simulink model "LoadLevel3_VF"  (R2023a)
settings: Solver=VariableStepAuto  StartTime=0.0  StopTime=250  RelTol=1e-3
undefined symbols (not defined in the file): a, Ac, Bc, Cc, D1, Dc, Delta, find_system, Fnom, gcbh, I21_init_imag, I21_init_real, Ibase1, Ibase2, Iw1A_init_mag, Iw1A_init_pha, Iw1B_init_mag, Iw1B_init_pha, Iw1C_init_mag, Iw1C_init_pha, Iw2A_init_mag, Iw2A_init_pha, Iw2B_init_mag, Iw2B_init_pha, Iw2C_init_mag, Iw2C_init_pha, j, kr, ks, Nmax, Pnom, psi, RegulatorDeadBand, RegulatorDelay, RegulatorVref, sps_rtmsupport, Vnom1, Vnom2, w, Z1pu, Z2pu, Ztpu
libraries: spsThreePhaseVIMeasurementLib x15, spsThreePhasePISectionLineLib x14, spsThreePhaseParallelRLCLoadLib x11, spsControlledCurrentSourceLib x6, spsThreePhaseTransformerTwoWindingsLib x5, spsThreePhaseBreakerLib x2, spsExcitationSystemLib x2, spsHydraulicTurbineandGovernorLib x2, spsSynchronousMachinepuStandardLib x2, spsThreePhaseSeriesRLCBranchLib x2, spsGroundLib x2, spsSequenceAnalyzerPhasorLib x1
(part 1 of 3)
settings Model: Creator=moham  LastModifiedBy=pipe1
settings SolverCC: AlgebraicLoopSolver=TrustRegion
settings DebuggingCC: ArithmeticOperatorsInVariantConditions=warning
settings SFSimCC: CustomCodeUndefinedFunction=UseInterfaceOnly

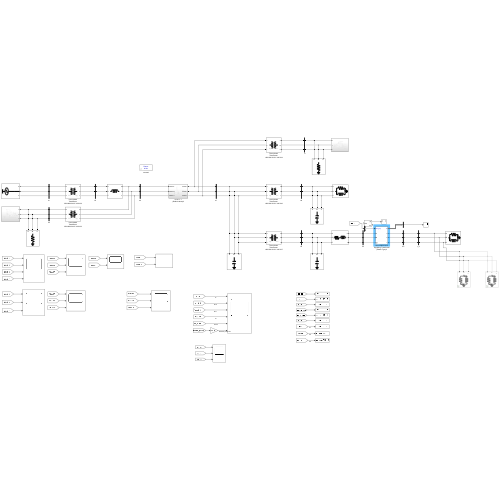
[thumbnail: Simulink's stored preview of the top-level diagram]
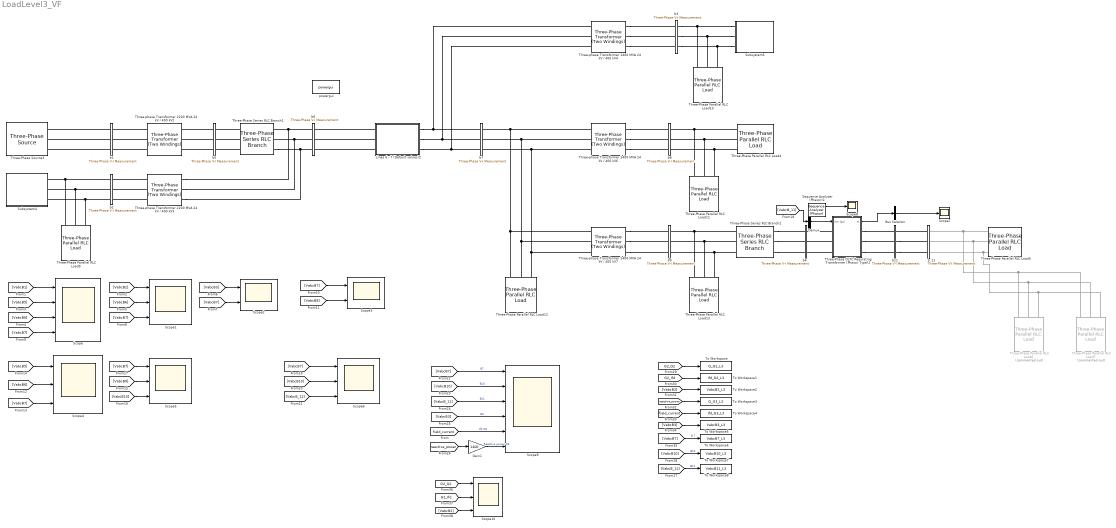
== system LoadLevel3_VF ==
  Bus Selector : BusSelector  OutputSignals=Tap  OutputAsBus=on
  Demux : Demux  Outputs=3
  Gain1 : Gain  Gain=1400
  Lines 6 - 7 (Default values)2 : Subsystem
  Scope : Scope  NumInputPorts=4
  Scope{1,4..6,10} (5 alike) : Scope  NumInputPorts=3
  Scope2 : Scope  NumInputPorts=2
  Scope3 : Scope  NumInputPorts=2
  Scope7 : Scope
  Scope8 : Scope
  Scope9 : Scope  NumInputPorts=6
  Sequence Analyzer (Phasor)2 : spsSequenceAnalyzerPhasorLib/Sequence Analyzer (Phasor)  seq=Positive
      settings: LibrarySourceBlock=|
      | sps_lib/Sensors and Measurements/Sequence Analyzer
      | (Phasor)
  Subsystem4 : Subsystem
  Subsystem5 : Subsystem
  Three-Phase Parallel RLC Load10 : spsThreePhaseParallelRLCLoadLib/Three-Phase Parallel RLC Load  LConnTagsString=A|B|C  Configuration=Y (grounded)  NominalVoltage=(24000)*1  Vabc=[1e3 1e3 1e3]  Vabcp=[1e3 1e3 1e3]  NominalFrequency=60  UnbalancedPower=off  ActivePower=500000000  InductivePower=0  CapacitivePower=0  Pabc=[10e3 9e3 11e3]  QLabc=[100 90 110]  QCabc=[100 90 110]  Pabcp=[10e3 9e3 11e3]  QLabcp=[100 90 110]  QCabcp=[100 90 110]  Measurements=None  LoadType=constant PQ
  Three-Phase Parallel RLC Load11 : spsThreePhaseParallelRLCLoadLib/Three-Phase Parallel RLC Load  LConnTagsString=A|B|C  Configuration=Y (grounded)  NominalVoltage=33000  Vabc=[1e3 1e3 1e3]  Vabcp=[1e3 1e3 1e3]  NominalFrequency=60  UnbalancedPower=off  ActivePower=0  InductivePower=0  CapacitivePower=600e6  Pabc=[10e3 9e3 11e3]  QLabc=[100 90 110]  QCabc=[100 90 110]  Pabcp=[10e3 9e3 11e3]  QLabcp=[100 90 110]  QCabcp=[100 90 110]  Measurements=None  LoadType=constant PQ
  Three-Phase Parallel RLC Load12 : spsThreePhaseParallelRLCLoadLib/Three-Phase Parallel RLC Load  LConnTagsString=A|B|C  Configuration=Y (grounded)  NominalVoltage=400e3  Vabc=[1e3 1e3 1e3]  Vabcp=[1e3 1e3 1e3]  NominalFrequency=60  UnbalancedPower=off  ActivePower=0  InductivePower=0  CapacitivePower=763e6  Pabc=[10e3 9e3 11e3]  QLabc=[100 90 110]  QCabc=[100 90 110]  Pabcp=[10e3 9e3 11e3]  QLabcp=[100 90 110]  QCabcp=[100 90 110]  Measurements=None  LoadType=constant PQ
  Three-Phase Parallel RLC Load13 : spsThreePhaseParallelRLCLoadLib/Three-Phase Parallel RLC Load  LConnTagsString=A|B|C  Configuration=Y (grounded)  NominalVoltage=33000  Vabc=[1e3 1e3 1e3]  Vabcp=[1e3 1e3 1e3]  NominalFrequency=60  UnbalancedPower=off  ActivePower=0  InductivePower=0  CapacitivePower=1710e6  Pabc=[10e3 9e3 11e3]  QLabc=[100 90 110]  QCabc=[100 90 110]  Pabcp=[10e3 9e3 11e3]  QLabcp=[100 90 110]  QCabcp=[100 90 110]  Measurements=None  LoadType=constant PQ
  Three-Phase Parallel RLC Load4 : spsThreePhaseParallelRLCLoadLib/Three-Phase Parallel RLC Load  LConnTagsString=A|B|C  Configuration=Y (grounded)  NominalVoltage=33000  Vabc=[1e3 1e3 1e3]  Vabcp=[1e3 1e3 1e3]  NominalFrequency=60  UnbalancedPower=off  ActivePower=3345e6  InductivePower=1038e6  CapacitivePower=0  Pabc=[10e3 9e3 11e3]  QLabc=[100 90 110]  QCabc=[100 90 110]  Pabcp=[10e3 9e3 11e3]  QLabcp=[100 90 110]  QCabcp=[100 90 110]  Measurements=None  LoadType=constant PQ
  Three-Phase Parallel RLC Load5 : spsThreePhaseParallelRLCLoadLib/Three-Phase Parallel RLC Load  LConnTagsString=A|B|C  Configuration=Y (grounded)  NominalVoltage=(11000)  Vabc=[1e3 1e3 1e3]  Vabcp=[1e3 1e3 1e3]  NominalFrequency=60  UnbalancedPower=off  ActivePower=3460e6  InductivePower=993e6  CapacitivePower=0  Pabc=[10e3 9e3 11e3]  QLabc=[100 90 110]  QCabc=[100 90 110]  Pabcp=[10e3 9e3 11e3]  QLabcp=[100 90 110]  QCabcp=[100 90 110]  Measurements=None  LoadType=constant PQ
  Three-Phase Parallel RLC Load6 : spsThreePhaseParallelRLCLoadLib/Three-Phase Parallel RLC Load  Commented=on  LConnTagsString=A|B|C  Configuration=Y (grounded)  NominalVoltage=11e3  Vabc=[1e3 1e3 1e3]  Vabcp=[1e3 1e3 1e3]  NominalFrequency=60  UnbalancedPower=off  ActivePower=3435e6/2  InductivePower=985e6/2  CapacitivePower=0  Pabc=[10e3 9e3 11e3]  QLabc=[100 90 110]  QCabc=[100 90 110]  Pabcp=[10e3 9e3 11e3]  QLabcp=[100 90 110]  QCabcp=[100 90 110]  Measurements=None  LoadType=constant Z
  Three-Phase Parallel RLC Load7 : spsThreePhaseParallelRLCLoadLib/Three-Phase Parallel RLC Load  Commented=on  LConnTagsString=A|B|C  Configuration=Y (grounded)  NominalVoltage=11e3  Vabc=[1e3 1e3 1e3]  Vabcp=[1e3 1e3 1e3]  NominalFrequency=60  UnbalancedPower=off  ActivePower=3435e6/2  InductivePower=985e6/2  CapacitivePower=0  Pabc=[10e3 9e3 11e3]  QLabc=[100 90 110]  QCabc=[100 90 110]  Pabcp=[10e3 9e3 11e3]  QLabcp=[100 90 110]  QCabcp=[100 90 110]  Measurements=None  LoadType=constant I
  Three-Phase Parallel RLC Load9 : spsThreePhaseParallelRLCLoadLib/Three-Phase Parallel RLC Load  LConnTagsString=A|B|C  Configuration=Y (grounded)  NominalVoltage=(24000)*1  Vabc=[1e3 1e3 1e3]  Vabcp=[1e3 1e3 1e3]  NominalFrequency=60  UnbalancedPower=off  ActivePower=500000000  InductivePower=0  CapacitivePower=0  Pabc=[10e3 9e3 11e3]  QLabc=[100 90 110]  QCabc=[100 90 110]  Pabcp=[10e3 9e3 11e3]  QLabcp=[100 90 110]  QCabcp=[100 90 110]  Measurements=None  LoadType=constant PQ
  Three-Phase Series RLC Branch1 : spsThreePhaseSeriesRLCBranchLib/Three-Phase Series RLC Branch  LConnTagsString=A|B|C  RConnTagsString=A|B|C  BranchType=L  Resistance=1  Inductance=0.016976  Capacitance=1e-6  Measurements=None
  Three-Phase Series RLC Branch2 : spsThreePhaseSeriesRLCBranchLib/Three-Phase Series RLC Branch  LConnTagsString=A|B|C  RConnTagsString=A|B|C  BranchType=RL  Resistance=0.01089  Inductance=8.666e-5  Capacitance=1e-6  Measurements=None
  Three-Phase OLTC Regulating Transformer (Phasor Type)2 : Subsystem  AncestorBlock=|  DialogController=POWERSYS.PowerSysDialog  LoadFcn=sps_rtmsupport('LoadFcn',gcbh); %find_system(gcs,'FollowLinks', 'on', 'LookUnderMasks', 'all');  StartFcn=sps_rtmsupport('StartFcn',gcbh);  StopFcn=sps_rtmsupport('StopFcn',gcbh);  mask(Three-Phase OLTC Regulating Transformer (Phasor Type)){Winding1Connection=Yg, Winding2Connection=Yg, PnomFnom=[4000e6,  60], Winding1=[33e3, 0, 0.04 ], Winding2=[11e3,  0, 0.04 ], Iw2_init=[0 , 0], RmXm=[500, 500], TapOnWinding=Winding 2, WindingTap=[ 0, 0.004], dU=0.00625, TapMinMax=[ -16, +16], InitialTap=0, TapSelectionTime=5, ExternalControl=off, RegulatorOn=on, Regulator=[0.895,  0.01, 0]}
      | sps_lib/Power Grid Elements/Three-Phase OLTC
      | Regulating Transformer
      | (Phasor Type)
      mask prompts: Winding1Connection "Winding 1 connection (ABC terminals):"; Winding2Connection "Winding 2 connection (abc terminals):"; PnomFnom "Nominal power and frequency [Pn(VA), fn(Hz)]"; Winding1 "Winding 1 parameters [V1 Ph-Ph(Vrms), R1(pu),  X1(pu)]"; Winding2 "Winding 2 parameters [V2 Ph-Ph(Vrms),  R2(pu),  X2(pu)]"; Iw2_init "Initial pos. seq. output currents of winding 2 [Mag(pu),  Phase(deg)]"; RmXm "Magnetization branch [Rm(pu)  Xm(pu)]"; TapOnWinding "OLTC on:"; WindingTap "Tapped regulation winding [Rt(pu),  Xt(pu)]"; dU "Voltage step per tap (pu)"; TapMinMax "Minimum and maximum tap positions [Min, Max]"; InitialTap "Initial tap position"; TapSelectionTime "Tap selection time (s)"; ExternalControl "External control of OLTC"; RegulatorOn "Voltage regulator"; Regulator "Regulator parameters [ Vref(pu) DeadBand(pu)  Delay(s)]"
      mask help: Implement phasor model of three-phase OLTC regulating transformer. It consists of two fixed windings and a third tapped winding (regulation winding) connected in series with either winding 1 or winding 2. Voltage ratio and transformer impedance vary with tap position. A +30 degrees or -30 degrees phase shift is introduced when winding 1 or winding 2 are connected in Delta.
      mask init:
      | [a,Z1pu,Z2pu,Ztpu,psi,ks,kr,RegulatorVref, RegulatorDeadBand,RegulatorDelay,Iw2A_init_mag,Iw2B_init_mag,Iw2C_init_mag, Iw2A_init_pha,Iw2B_init_pha,Iw2C_init_pha,N2_N1,Iw1A_init_mag,Iw1B_init_mag,Iw1C_init_mag,Iw1A_init_pha,Iw1B_init_pha,Iw1C_init_pha,I21_init_real,I21_init_imag,Nmax,w,Vnom1,Vnom2,Ibase1,Ibase2,Pnom,Fnom ] = powericon('OLTCRegulatingTansformerInit',InitialTap, TapMinMax,PnomFnom,Winding1,Winding1Connection,Winding2,Winding2Connection,Regulator,Iw2_init,TapOnWinding,dU,WindingTap);
      | OLTCtransformerCback(gcbh,2);
      | power_initmask();
      settings: CopyFcn=sps_rtmsupport('CopyFcn',gcbh);  DeleteFcn=sps_rtmsupport('DeleteFcn',gcbh);  UndoDeleteFcn=sps_rtmsupport('UndoDeleteFcn',gcbh);  ModelCloseFcn=sps_rtmsupport('ModelCloseFcn',gcbh);  PreSaveFcn=sps_rtmsupport('PreSaveFcn',gcbh);  PostSaveFcn=sps_rtmsupport('PostSaveFcn',gcbh);  NameChangeFcn=sps_rtmsupport('NameChangeFcn',gcbh);  PreCopyFcn=sps_rtmsupport('PreCopyFcn',gcbh);  OpenFcn=sps_rtmsupport('OpenFcn',gcbh, [1 2 8 14 15]);  CloseFcn=sps_rtmsupport('CloseFcn',gcbh);  PreDeleteFcn=sps_rtmsupport('PreDeleteFcn',gcbh);
      mask Help: helpview(psbhelp)
      mask TypeOptions Winding1Connection: Y | Yg | Delta (D1) | Delta (D11)
      mask TypeOptions Winding2Connection: Y | Yg | Delta (D1) | Delta (D11)
      mask TypeOptions TapOnWinding: Winding 1 | Winding 2
      mask Callback ExternalControl: %OLTCtransformerCback(gcbh,2);
      mask TypeOptions RegulatorOn: off | on
      mask Callback RegulatorOn: OLTCtransformerCback(gcbh,3);
      mask DialogControl Transformerparameters Prompt: Transformer
      mask DialogControl OLTCandVoltageRegulatorparameters Prompt: OLTC and Voltage Regulator
      mask Display: disp('')
  Three-Phase Source3 : spsThreePhaseSourceLib/Three-Phase Source  InternalConnection=Yg  VoltagePhases=off  Voltage=(24000)*0.98  PhaseAngle=0  Voltage_phases=[25e3 25e3 25e3]/sqrt(3)  PhaseAngles_phases=[0 -120 +120]  Frequency=60  NonIdealSource=off  SpecifyImpedance=off  Resistance=0.8929  Inductance=16.58e-3  ShortCircuitLevel=100e6  BaseVoltage=24e3  XRratio=7  BusType=swing  Pref=50000000000  Qref=0  Prefabc=[10e3, 10e3, 10e3]  Qrefabc=[0, 0, 0]  Qmin=-Inf  Qmax=Inf
  Three-phase Transformer 1400 MVA 24 kV / 400 kV4 : spsThreePhaseTransformerTwoWindingsLib/Three-Phase Transformer (Two Windings)  Winding1Connection=Delta (D1)  Winding2Connection=Yg  CoreType=Three single-phase transformers  SetSaturation=off  Hysteresis=off  DataFile='hysteresis'  SetInitialFlux=off  Measurements=None  UNITS=pu  NominalPower=[ 1400e6 60 ]  Winding1="[ 24e3 0  0.175/2]"  Winding2=[ 400e3/0.9024 0 0.175/2]  Rm=500  Lm=500  L0=0.5  Saturation="[ 0,0  ;  0.005,1.2  ;  1.0,1.4 ]"  InitialFluxes=[ 0.8 , -0.8 , 0.7 ]  BreakLoop=off  DiscreteSolver=Trapezoidal iterative  DataType=off  TransfoNumber=0
  Three-phase Transformer 1400 MVA 24 kV / 400 kV6 : spsThreePhaseTransformerTwoWindingsLib/Three-Phase Transformer (Two Windings)  Winding1Connection=Yg  Winding2Connection=Delta (D1)  CoreType=Three single-phase transformers  SetSaturation=off  Hysteresis=off  DataFile='hysteresis'  SetInitialFlux=off  Measurements=None  UNITS=pu  NominalPower=[ 4000e6 60 ]  Winding1="[ 400e3 0  0.12/2]"  Winding2=[ 33e3/1.0664 0 0.12/2]  Rm=500  Lm=500  L0=0.5  Saturation="[ 0,0  ;  0.005,1.2  ;  1.0,1.4 ]"  InitialFluxes=[ 0.8 , -0.8 , 0.7 ]  BreakLoop=off  DiscreteSolver=Trapezoidal iterative  DataType=off  TransfoNumber=0
  Three-phase Transformer 1400 MVA 24 kV / 400 kV7 : spsThreePhaseTransformerTwoWindingsLib/Three-Phase Transformer (Two Windings)  Winding1Connection=Yg  Winding2Connection=Delta (D1)  CoreType=Three single-phase transformers  SetSaturation=off  Hysteresis=off  DataFile='hysteresis'  SetInitialFlux=off  Measurements=None  UNITS=pu  NominalPower=[ 4000e6 60 ]  Winding1="[ 400e3 0  0.104/2]"  Winding2=[ 33e3/1.08 0 0.104/2]  Rm=500  Lm=500  L0=0.5  Saturation="[ 0,0  ;  0.005,1.2  ;  1.0,1.4 ]"  InitialFluxes=[ 0.8 , -0.8 , 0.7 ]  BreakLoop=off  DiscreteSolver=Trapezoidal iterative  DataType=off  TransfoNumber=0
  Three-phase Transformer 2200 MVA 24 kV / 400 kV2 : spsThreePhaseTransformerTwoWindingsLib/Three-Phase Transformer (Two Windings)  Winding1Connection=Delta (D1)  Winding2Connection=Yg  CoreType=Three single-phase transformers  SetSaturation=off  Hysteresis=off  DataFile='hysteresis'  SetInitialFlux=off  Measurements=None  UNITS=pu  NominalPower=[ 7000e6 60 ]  Winding1="[ 24e3 0  0.14/2]"  Winding2=[ 400e3/0.8857 0 0.14/2]  Rm=1000  Lm=1000  L0=0.5  Saturation="[ 0,0  ;  0.005,1.2  ;  1.0,1.4 ]"  InitialFluxes=[ 0.8 , -0.8 , 0.7 ]  BreakLoop=off  DiscreteSolver=Trapezoidal iterative  DataType=off  TransfoNumber=0
  Three-phase Transformer 2200 MVA 24 kV / 400 kV3 : spsThreePhaseTransformerTwoWindingsLib/Three-Phase Transformer (Two Windings)  Winding1Connection=Delta (D1)  Winding2Connection=Yg  CoreType=Three single-phase transformers  SetSaturation=off  Hysteresis=off  DataFile='hysteresis'  SetInitialFlux=off  Measurements=None  UNITS=pu  NominalPower=[ 2200e6 60 ]  Winding1="[ 24e3 0  0.099/2]"  Winding2=[ 400e3/0.8857 0 0.099/2]  Rm=500  Lm=500  L0=0.5  Saturation="[ 0,0  ;  0.005,1.2  ;  1.0,1.4 ]"  InitialFluxes=[ 0.8 , -0.8 , 0.7 ]  BreakLoop=off  DiscreteSolver=Trapezoidal iterative  DataType=off  TransfoNumber=0
  To Workspace : ToWorkspace  VariableName=Q_G2_L3  SaveFormat=Timeseries  SampleTime=-1
  To Workspace1 : ToWorkspace  VariableName=Ifd_G2_L3  SaveFormat=Timeseries  SampleTime=-1
  To Workspace2 : ToWorkspace  VariableName=VabcB2_L3  SaveFormat=Timeseries  SampleTime=-1
  To Workspace3 : ToWorkspace  VariableName=Q_G3_L3  SaveFormat=Timeseries  SampleTime=-1
  To Workspace4 : ToWorkspace  VariableName=Ifd_G3_L3  SaveFormat=Timeseries  SampleTime=-1
  To Workspace5 : ToWorkspace  VariableName=VabcB3_L3  SaveFormat=Timeseries  SampleTime=-1
  To Workspace6 : ToWorkspace  VariableName=VabcB7_L3  SaveFormat=Timeseries  SampleTime=-1
  To Workspace7 : ToWorkspace  VariableName=VabcB10_L3  SaveFormat=Timeseries  SampleTime=-1
  To Workspace8 : ToWorkspace  VariableName=VabcB11_L3  SaveFormat=Timeseries  SampleTime=-1
  b1 : spsThreePhaseVIMeasurementLib/Three-Phase V-I Measurement  VoltageMeasurement=phase-to-ground  SetLabelV=on  LabelV=VabcB1  Vpu=on  VpuLL=off  CurrentMeasurement=yes  SetLabelI=on  LabelI=IabcB1  Ipu=on  Pbase=4000e6  Vbase=24e3  OutputType=Magnitude  PhasorSimulation=on  PSBequivalent=0
  b11 : spsThreePhaseVIMeasurementLib/Three-Phase V-I Measurement  VoltageMeasurement=phase-to-ground  SetLabelV=on  LabelV=VabcB11  Vpu=on  VpuLL=off  CurrentMeasurement=yes  SetLabelI=on  LabelI=IabcB11  Ipu=on  Pbase=4000e6  Vbase=11e3  OutputType=Complex  PhasorSimulation=on  PSBequivalent=0
  b2 : spsThreePhaseVIMeasurementLib/Three-Phase V-I Measurement  VoltageMeasurement=phase-to-ground  SetLabelV=on  LabelV=VabcB2  Vpu=on  VpuLL=off  CurrentMeasurement=yes  SetLabelI=on  LabelI=IabcB2  Ipu=on  Pbase=2200e6  Vbase=24e3  OutputType=Magnitude  PhasorSimulation=on  PSBequivalent=0
  b3 : spsThreePhaseVIMeasurementLib/Three-Phase V-I Measurement  VoltageMeasurement=phase-to-ground  SetLabelV=on  LabelV=VabcB3  Vpu=on  VpuLL=off  CurrentMeasurement=yes  SetLabelI=on  LabelI=IabcB3  Ipu=on  Pbase=1100e6  Vbase=24e3  OutputType=Magnitude  PhasorSimulation=on  PSBequivalent=0
  b4 : spsThreePhaseVIMeasurementLib/Three-Phase V-I Measurement  VoltageMeasurement=phase-to-ground  SetLabelV=on  LabelV=VabcB10  Vpu=on  VpuLL=off  CurrentMeasurement=yes  SetLabelI=on  LabelI=IabcB10  Ipu=on  Pbase=4000e6  Vbase=33e3  OutputType=Magnitude  PhasorSimulation=on  PSBequivalent=0
  b5 : spsThreePhaseVIMeasurementLib/Three-Phase V-I Measurement  VoltageMeasurement=phase-to-ground  SetLabelV=on  LabelV=VabcB5  Vpu=on  VpuLL=off  CurrentMeasurement=yes  SetLabelI=on  LabelI=IabcB5  Ipu=on  Pbase=4000e6  Vbase=400e3  OutputType=Magnitude  PhasorSimulation=on  PSBequivalent=0
  b6 : spsThreePhaseVIMeasurementLib/Three-Phase V-I Measurement  VoltageMeasurement=phase-to-ground  SetLabelV=on  LabelV=VabcB6  Vpu=on  VpuLL=off  CurrentMeasurement=yes  SetLabelI=on  LabelI=IabcB6  Ipu=on  Pbase=4000e6  Vbase=400e3  OutputType=Magnitude  PhasorSimulation=on  PSBequivalent=0
  b7 : spsThreePhaseVIMeasurementLib/Three-Phase V-I Measurement  VoltageMeasurement=phase-to-ground  SetLabelV=on  LabelV=VabcB7  Vpu=on  VpuLL=off  CurrentMeasurement=yes  SetLabelI=on  LabelI=IabcB7  Ipu=on  Pbase=4000e6  Vbase=400e3  OutputType=Magnitude  PhasorSimulation=on  PSBequivalent=0
  b8 : spsThreePhaseVIMeasurementLib/Three-Phase V-I Measurement  VoltageMeasurement=phase-to-ground  SetLabelV=on  LabelV=VabcB8  Vpu=on  VpuLL=off  CurrentMeasurement=yes  SetLabelI=on  LabelI=IabcB8  Ipu=on  Pbase=4000e6  Vbase=33e3  OutputType=Magnitude  PhasorSimulation=on  PSBequivalent=0
  b9 : spsThreePhaseVIMeasurementLib/Three-Phase V-I Measurement  VoltageMeasurement=phase-to-ground  SetLabelV=on  LabelV=VabcB9  Vpu=on  VpuLL=off  CurrentMeasurement=yes  SetLabelI=on  LabelI=IabcB9  Ipu=on  Pbase=4000e6  Vbase=33e3  OutputType=Magnitude  PhasorSimulation=on  PSBequivalent=0
  b_11 : spsThreePhaseVIMeasurementLib/Three-Phase V-I Measurement  VoltageMeasurement=phase-to-ground  SetLabelV=on  LabelV=VabcB_11  Vpu=on  VpuLL=off  CurrentMeasurement=yes  SetLabelI=on  LabelI=IabcB_11  Ipu=on  Pbase=4000e6  Vbase=11e3  OutputType=Magnitude  PhasorSimulation=on  PSBequivalent=0
  powergui : sps_lib/powergui  Priority=1  SimulationMode=Phasor  SampleTime=5e-6  frequency=60  Iterations=50  frequencyindice=60  Pbase=100e6  ErrMax=1e-4  UnitsV=kV  UnitsW=MW  buscounter=0  FunctionMessages=off  echomessages=off  EnableUseOfTLC=off  CurrentSourceSwitches=off  DisableSnubberDevices=off  DisableRonSwitches=off  DisableVfSwitches=off  DisplayEquations=off  AutomaticDiscreteSolvers=off  SolverType=Tustin/Backward Euler (TBE)  Interpol=off  ExternalGateDelay=off  methode=off  Ts=100  x0status=blocks  SPID=on  SwTol=0  HookPort=off  NonlinearTolerance=1e-4  nMaxIteration=100  ContinueOnMaxIteration=off  RestoreLinks=warning  ResistiveCurrentMeasurement=off  Frange=[0:2:500]  Ylog=off  Xlog=on  ShowGrid=off  save=off  variable=ZData  structure=0  ZoomFFT=off  StartTime=0.0  cycles=1  DisplayStyle=1  fundamental=60  FreqAxis=off  MaxFrequency=1000  frequencyindicesteady=1  RmsSteady=1  display=off
  wires:
  [VabcB7] -> Scope6/1
  [VabcB10] -> Scope6/2
  [VabcB7] -> Scope5/1
  [VabcB7] -> Scope2/2
  [VabcB2] -> Scope1/1
  [VabcB10] -> Scope5/3
  [VabcB3] -> Scope2/1
  [VabcB5] -> Scope4/1
  [VabcB9] -> Scope5/2
  [VabcB5] -> Scope/2
  [VabcB7] -> Scope4/3
  [VabcB6] -> Scope4/2
  [VabcB7] -> Scope3/1
  [VabcB7] -> Scope1/3
  [VabcB_11] -> Scope6/3
  [VabcB1] -> Scope/1
  [VabcB6] -> Scope1/2
  [VabcB8] -> Scope3/2
  [VabcB6] -> Scope/3
  [VabcB7] -> Scope/4
  [VabcB_11] -> Demux/1
  Sequence Analyzer (Phasor)2/1 -> Scope8/1
  Bus Selector/1 -> Scope7/1
  Three-Phase OLTC Regulating Transformer (Phasor Type)2/1(m) -> Bus Selector/1
  Demux/2 -> Three-Phase OLTC Regulating Transformer (Phasor Type)2/1(Vm (pu))
  [reactive_power] -> To Workspace3/1
  [VabcB2] -> Scope10/3
  [G2_Q2] -> Scope10/1
  [G2_Ifd] -> Scope10/2
  [VabcB7] -> To Workspace6/1  "B 7"
  Gain1/1 -> Scope9/6  "Reactive power G3"
  [VabcB2] -> To Workspace2/1
  [field_current] -> To Workspace4/1
  [VabcB3] -> To Workspace5/1
  [VabcB10] -> To Workspace7/1  "B10"
  [G2_Q2] -> To Workspace/1
  [VabcB_11] -> Scope9/3  "B11"
  [reactive_power] -> Gain1/1
  [VabcB10] -> Scope9/2  "B10"
  [VabcB3] -> Scope9/4  "B3"
  [G2_Ifd] -> To Workspace1/1
  [VabcB_11] -> To Workspace8/1  "B11"
  [VabcB7] -> Scope9/1  "B7"
  [field_current] -> Scope9/5  "Ifd G3"
  connections:
  Three-phase Transformer 1400 MVA 24 kV / 400 kV6/LConn1 -- Three-Phase Parallel RLC Load12/LConn1 -- Three-phase Transformer 1400 MVA 24 kV / 400 kV7/LConn1 -- b7/RConn1
  Three-phase Transformer 2200 MVA 24 kV / 400 kV3/RConn1 -- b6/LConn1 -- Three-Phase Series RLC Branch1/RConn1
  Subsystem5/RConn2 -- Three-Phase Parallel RLC Load10/LConn2 -- b3/LConn2
  Three-Phase Parallel RLC Load13/LConn3 -- Three-Phase Series RLC Branch2/LConn3 -- b9/RConn3
  Three-phase Transformer 2200 MVA 24 kV / 400 kV3/RConn2 -- b6/LConn2 -- Three-Phase Series RLC Branch1/RConn2
  b7/RConn2 -- Three-Phase Parallel RLC Load12/LConn2 -- Three-phase Transformer 1400 MVA 24 kV / 400 kV7/LConn2 -- Three-phase Transformer 1400 MVA 24 kV / 400 kV6/LConn2
  Lines 6 - 7 (Default values)2/RConn2 -- Three-phase Transformer 1400 MVA 24 kV / 400 kV4/RConn2 -- b7/LConn2
  Three-Phase Series RLC Branch1/RConn3 -- Three-phase Transformer 2200 MVA 24 kV / 400 kV3/RConn3 -- b6/LConn3
  b7/RConn3 -- Three-Phase Parallel RLC Load12/LConn3 -- Three-phase Transformer 1400 MVA 24 kV / 400 kV7/LConn3 -- Three-phase Transformer 1400 MVA 24 kV / 400 kV6/LConn3
  b9/RConn1 -- Three-Phase Parallel RLC Load13/LConn1 -- Three-Phase Series RLC Branch2/LConn1
  Three-Phase Parallel RLC Load9/LConn3 -- b2/LConn3 -- Subsystem4/RConn3
  Three-Phase Parallel RLC Load9/LConn1 -- b2/LConn1 -- Subsystem4/RConn1
  Lines 6 - 7 (Default values)2/RConn1 -- Three-phase Transformer 1400 MVA 24 kV / 400 kV4/RConn1 -- b7/LConn1
  Subsystem5/RConn3 -- b3/LConn3 -- Three-Phase Parallel RLC Load10/LConn3
  Subsystem5/RConn1 -- Three-Phase Parallel RLC Load10/LConn1 -- b3/LConn1
  Three-Phase Parallel RLC Load9/LConn2 -- b2/LConn2 -- Subsystem4/RConn2
  b8/RConn2 -- Three-Phase Parallel RLC Load4/LConn2 -- Three-Phase Parallel RLC Load11/LConn2
  b8/RConn1 -- Three-Phase Parallel RLC Load4/LConn1 -- Three-Phase Parallel RLC Load11/LConn1
  Lines 6 - 7 (Default values)2/RConn3 -- Three-phase Transformer 1400 MVA 24 kV / 400 kV4/RConn3 -- b7/LConn3
  b9/RConn2 -- Three-Phase Parallel RLC Load13/LConn2 -- Three-Phase Series RLC Branch2/LConn2
  b8/RConn3 -- Three-Phase Parallel RLC Load4/LConn3 -- Three-Phase Parallel RLC Load11/LConn3
  Three-phase Transformer 1400 MVA 24 kV / 400 kV4/LConn1 -- b3/RConn1
  Three-phase Transformer 2200 MVA 24 kV / 400 kV2/LConn3 -- b1/RConn3
  b5/LConn3 -- Three-phase Transformer 2200 MVA 24 kV / 400 kV2/RConn3
  Three-phase Transformer 1400 MVA 24 kV / 400 kV7/RConn2 -- b9/LConn2
  Three-phase Transformer 1400 MVA 24 kV / 400 kV6/RConn3 -- b8/LConn3
  Three-Phase Series RLC Branch1/LConn2 -- b5/RConn2
  Three-phase Transformer 1400 MVA 24 kV / 400 kV4/LConn3 -- b3/RConn3
  Three-phase Transformer 1400 MVA 24 kV / 400 kV4/LConn2 -- b3/RConn2
  Three-Phase Series RLC Branch1/LConn1 -- b5/RConn1
  b5/LConn1 -- Three-phase Transformer 2200 MVA 24 kV / 400 kV2/RConn1
  Lines 6 - 7 (Default values)2/LConn2 -- b6/RConn2
  Three-phase Transformer 2200 MVA 24 kV / 400 kV3/LConn1 -- b2/RConn1
  Three-phase Transformer 2200 MVA 24 kV / 400 kV2/LConn1 -- b1/RConn1
  b1/LConn1 -- Three-Phase Source3/RConn1
  Lines 6 - 7 (Default values)2/LConn3 -- b6/RConn3
  Three-phase Transformer 1400 MVA 24 kV / 400 kV6/RConn1 -- b8/LConn1
  Three-Phase Series RLC Branch1/LConn3 -- b5/RConn3
  b1/LConn2 -- Three-Phase Source3/RConn2
  Three-phase Transformer 2200 MVA 24 kV / 400 kV3/LConn2 -- b2/RConn2
  Three-phase Transformer 1400 MVA 24 kV / 400 kV6/RConn2 -- b8/LConn2
  Three-phase Transformer 2200 MVA 24 kV / 400 kV2/LConn2 -- b1/RConn2
  Three-phase Transformer 1400 MVA 24 kV / 400 kV7/RConn1 -- b9/LConn1
  b1/LConn3 -- Three-Phase Source3/RConn3
  Three-phase Transformer 2200 MVA 24 kV / 400 kV3/LConn3 -- b2/RConn3
  Lines 6 - 7 (Default values)2/LConn1 -- b6/RConn1
  Three-phase Transformer 1400 MVA 24 kV / 400 kV7/RConn3 -- b9/LConn3
  b5/LConn2 -- Three-phase Transformer 2200 MVA 24 kV / 400 kV2/RConn2
  Three-Phase Series RLC Branch2/RConn1 -- b4/LConn1
  Three-Phase Series RLC Branch2/RConn3 -- b4/LConn3
  Three-Phase Series RLC Branch2/RConn2 -- b4/LConn2
  b11/RConn2 -- b_11/LConn2
  Three-Phase OLTC Regulating Transformer (Phasor Type)2/LConn1 -- b4/RConn1
  Three-Phase OLTC Regulating Transformer (Phasor Type)2/RConn3 -- b11/LConn3
  b_11/LConn1 -- b11/RConn1
  Three-Phase OLTC Regulating Transformer (Phasor Type)2/RConn1 -- b11/LConn1
  Three-Phase OLTC Regulating Transformer (Phasor Type)2/LConn2 -- b4/RConn2
  Three-Phase OLTC Regulating Transformer (Phasor Type)2/LConn3 -- b4/RConn3
  Three-Phase OLTC Regulating Transformer (Phasor Type)2/RConn2 -- b11/LConn2
  b11/RConn3 -- b_11/LConn3
  Three-Phase Parallel RLC Load7/LConn2 -- b_11/RConn2 -- Three-Phase Parallel RLC Load5/LConn2 -- Three-Phase Parallel RLC Load6/LConn2
  Three-Phase Parallel RLC Load7/LConn3 -- b_11/RConn3 -- Three-Phase Parallel RLC Load5/LConn3 -- Three-Phase Parallel RLC Load6/LConn3
  Three-Phase Parallel RLC Load7/LConn1 -- b_11/RConn1 -- Three-Phase Parallel RLC Load5/LConn1 -- Three-Phase Parallel RLC Load6/LConn1

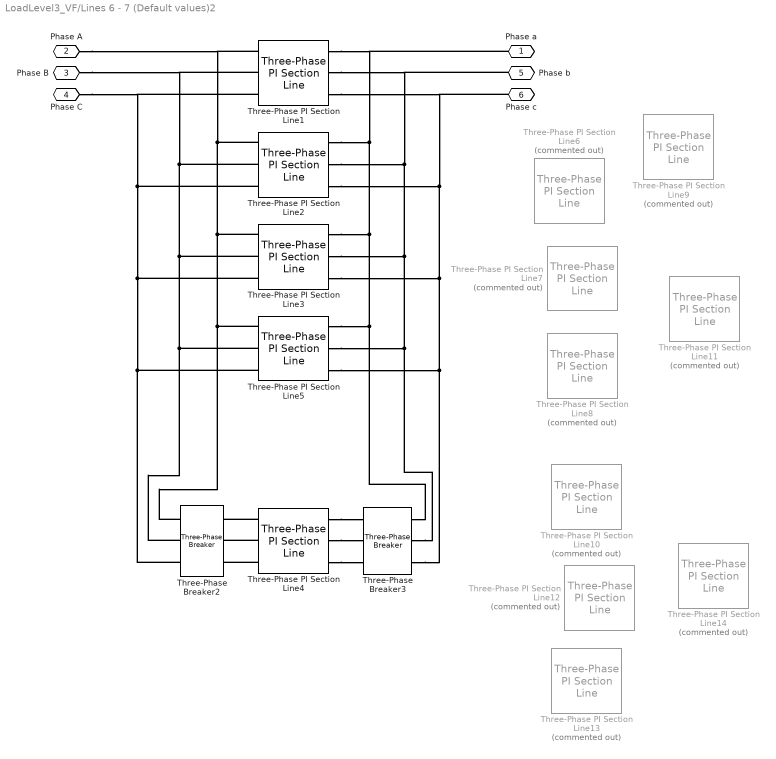
== system LoadLevel3_VF/Lines 6 - 7 (Default values)2 ==
  Three-Phase PI Section Line{1..5} (5 alike) : spsThreePhasePISectionLineLib/Three-Phase PI Section Line  LConnTagsString=a|b|c  RConnTagsString=A|B|C  Length=1.5  Frequency=60  Resistances=[2.4 2.4*3]  Inductances=[0.1222 0.1222*3]  Capacitances=[1.9447e-06 1.9447e-06*0.6]
  Three-Phase PI Section Line10 : spsThreePhasePISectionLineLib/Three-Phase PI Section Line  Commented=on  LConnTagsString=a|b|c  RConnTagsString=A|B|C  Length=15  Frequency=60  Resistances=[ 0.15 3*0.15] *10 /10  Inductances="[15e-3  3*0.0072]*10 /10"  Capacitances=[23.4e-6 70e-6]/(50*2)
  Three-Phase PI Section Line11 : spsThreePhasePISectionLineLib/Three-Phase PI Section Line  Commented=on  LConnTagsString=a|b|c  RConnTagsString=A|B|C  Length=10  Frequency=60  Resistances=[ 0.15 3*0.15] *10 /10  Inductances="[15e-3  3*0.0072]*10 /10"  Capacitances=[23.4e-6 70e-6]/(50*2)
  Three-Phase PI Section Line12 : spsThreePhasePISectionLineLib/Three-Phase PI Section Line  Commented=on  LConnTagsString=a|b|c  RConnTagsString=A|B|C  Length=10  Frequency=60  Resistances=[ 2.4 3*2.4] *5 /10  Inductances="[122e-3  3*0.122]*5 /10"  Capacitances=[1.95e-6 1.95e-6*0.6]/(5*10)
  Three-Phase PI Section Line13 : spsThreePhasePISectionLineLib/Three-Phase PI Section Line  Commented=on  LConnTagsString=a|b|c  RConnTagsString=A|B|C  Length=1  Frequency=60  Resistances=[2.4 2.4*3]  Inductances=[0.1222 0.1222*3]  Capacitances=[1.9447e-06 1.9447e-06*0.6]
  Three-Phase PI Section Line14 : spsThreePhasePISectionLineLib/Three-Phase PI Section Line  Commented=on  LConnTagsString=a|b|c  RConnTagsString=A|B|C  Length=10  Frequency=60  Resistances=[ 2.4 3*2.4] *5 /10  Inductances="[122e-3  3*0.122]*5 /10"  Capacitances=[1.95e-6 1.95e-6*0.6]/(5*10)
  Three-Phase PI Section Line6 : spsThreePhasePISectionLineLib/Three-Phase PI Section Line  Commented=on  LConnTagsString=a|b|c  RConnTagsString=A|B|C  Length=10  Frequency=60  Resistances=[ 1e-6*3.75*5/10 3*1e-6*3.75*5/10]  Inductances="[5*1e-6*7.2/10  3*5*1e-6*7.2/10]"  Capacitances=[300*1e-6/50 3*300*1e-6/50]
  Three-Phase PI Section Line7 : spsThreePhasePISectionLineLib/Three-Phase PI Section Line  Commented=on  LConnTagsString=a|b|c  RConnTagsString=A|B|C  Length=10  Frequency=60  Resistances=[ 2e-3*0.4*5*120*pi/10 3*2e-3*0.4*5*120*pi/10]  Inductances="[5*2e-3*7.2/10  3*5*2e-3*7.2/10]"  Capacitances=[300*2e-3/50 3*300*2e-3/50]
  Three-Phase PI Section Line8 : spsThreePhasePISectionLineLib/Three-Phase PI Section Line  Commented=on  LConnTagsString=a|b|c  RConnTagsString=A|B|C  Length=10  Frequency=60  Resistances=[ 0.15 3*0.15] *5 /10  Inductances="[7.2e-3  3*0.0072]*5 /10"  Capacitances=[23.4e-6 70e-6]/50
  Three-Phase PI Section Line9 : spsThreePhasePISectionLineLib/Three-Phase PI Section Line  Commented=on  LConnTagsString=a|b|c  RConnTagsString=A|B|C  Length=10  Frequency=60  Resistances=[ 0.15 3*0.15] *10 /10  Inductances="[7.2e-3  3*0.0072]*10 /10"  Capacitances=[23.4e-6 70e-6]/(50*2)
  Three-Phase Breaker2 : spsThreePhaseBreakerLib/Three-Phase Breaker  InitialState=closed  SwitchA=on  SwitchB=on  SwitchC=on  SwitchTimes="[10  300]"  External=off  BreakerResistance=0.01  SnubberResistance=1e6  SnubberCapacitance=inf  Measurements=None
  Three-Phase Breaker3 : spsThreePhaseBreakerLib/Three-Phase Breaker  InitialState=closed  SwitchA=on  SwitchB=on  SwitchC=on  SwitchTimes="[10  300]"  External=off  BreakerResistance=0.01  SnubberResistance=1e6  SnubberCapacitance=inf  Measurements=None
  Phase a : PMIOPort  Side=Right
  Phase A : PMIOPort  Port=2  Side=Left
  Phase B : PMIOPort  Port=3  Side=Left
  Phase C : PMIOPort  Port=4  Side=Left
  Phase b : PMIOPort  Port=5  Side=Right
  Phase c : PMIOPort  Port=6  Side=Right
  connections:
  Three-Phase Breaker2/LConn1 -- Three-Phase PI Section Line5/LConn1 -- Three-Phase PI Section Line3/LConn1 -- Three-Phase PI Section Line2/LConn1 -- Three-Phase PI Section Line1/LConn1 -- Phase A/RConn1
  Three-Phase Breaker2/LConn2 -- Three-Phase PI Section Line5/LConn2 -- Three-Phase PI Section Line3/LConn2 -- Three-Phase PI Section Line2/LConn2 -- Three-Phase PI Section Line1/LConn2 -- Phase B/RConn1
  Three-Phase Breaker2/LConn3 -- Three-Phase PI Section Line5/LConn3 -- Three-Phase PI Section Line3/LConn3 -- Three-Phase PI Section Line2/LConn3 -- Three-Phase PI Section Line1/LConn3 -- Phase C/RConn1
  Three-Phase Breaker3/RConn1 -- Three-Phase PI Section Line5/RConn1 -- Three-Phase PI Section Line3/RConn1 -- Three-Phase PI Section Line2/RConn1 -- Three-Phase PI Section Line1/RConn1 -- Phase a/RConn1
  Three-Phase Breaker3/RConn2 -- Three-Phase PI Section Line5/RConn2 -- Three-Phase PI Section Line3/RConn2 -- Three-Phase PI Section Line2/RConn2 -- Three-Phase PI Section Line1/RConn2 -- Phase b/RConn1
  Three-Phase Breaker3/RConn3 -- Three-Phase PI Section Line5/RConn3 -- Three-Phase PI Section Line3/RConn3 -- Three-Phase PI Section Line2/RConn3 -- Three-Phase PI Section Line1/RConn3 -- Phase c/RConn1
  Three-Phase PI Section Line4/RConn2 -- Three-Phase Breaker3/LConn2
  Three-Phase PI Section Line4/RConn3 -- Three-Phase Breaker3/LConn3
  Three-Phase PI Section Line4/LConn3 -- Three-Phase Breaker2/RConn3
  Three-Phase PI Section Line4/RConn1 -- Three-Phase Breaker3/LConn1
  Three-Phase PI Section Line4/LConn1 -- Three-Phase Breaker2/RConn1
  Three-Phase PI Section Line4/LConn2 -- Three-Phase Breaker2/RConn2

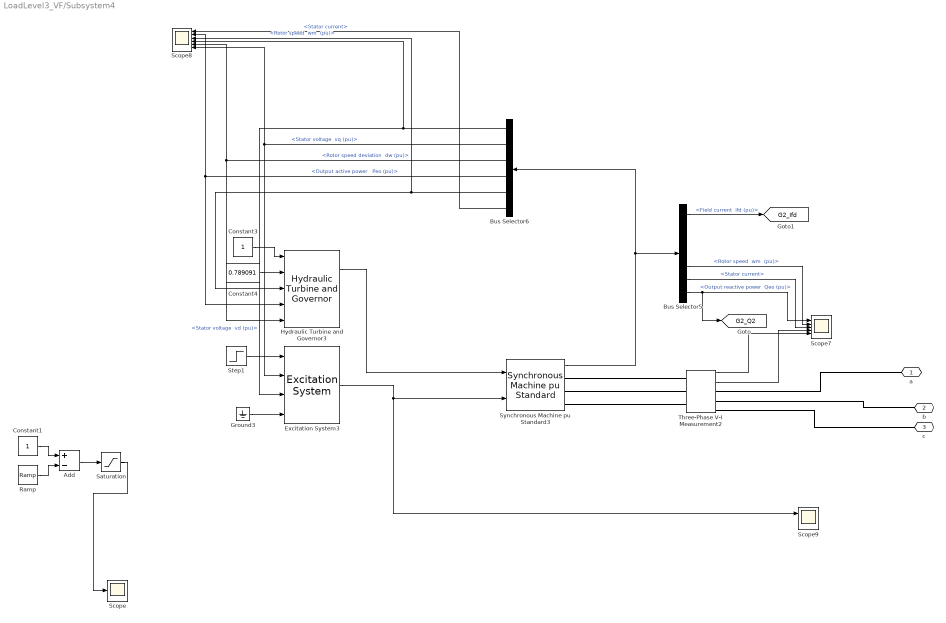
== system LoadLevel3_VF/Subsystem4 ==
  Add : Sum  Inputs=+-
  Bus Selector5 : BusSelector  OutputSignals="dq0 components.Field current  ifd (pu),dq0 components.Stator voltage  vd (pu),dq0 components.Stator voltage  vq (pu),Output active power   Peo (pu),Mechanical.Rotor speed  wm  (pu),Stator current,Output reactive power  Qeo (pu)"
  Bus Selector6 : BusSelector  OutputSignals="dq0 components.Stator voltage  vd (pu),dq0 components.Stator voltage  vq (pu),Mechanical.Rotor speed deviation  dw (pu),Output active power   Peo (pu),Mechanical.Rotor speed  wm  (pu),Stator current"
  Constant1 : Constant
  Constant3 : Constant
  Constant4 : Constant  Value=0.789091
  Excitation System3 : spsExcitationSystemLib/Excitation System  tr=20e-3  reg=[ 400, 0.02 ]  exc=[ 1, 0 ]  tgr=[ 0, 0 ]  damp=[ 0.001, 0.1 ]  sat=[ 0, 0 ]  lim=[ -11.5, 11.5, 0 ]  v0=[0.9646,1.69595]
      settings: LibrarySourceBlock=sps_lib/Electrical Machines/Synchronous Machine Control/Excitation System
  Ground3 : Ground
  Hydraulic Turbine and Governor3 : spsHydraulicTurbineandGovernorLib/Hydraulic Turbine and Governor  sm="[ 10/3  0.07 ]"  gate="[  0.01  0.97518  -0.1  0.1 ]"  reg="[  0.05  1.163  0.105  0  0.01  ]"  hyd="[  0  2.67  ]"  dref=0  po=0.793058
      settings: LibrarySourceBlock=|
      | sps_lib/Electrical Machines/Synchronous Machine Control/Hydraulic Turbine
      | and Governor
  Ramp : simulink/Sources/Ramp  slope=0.0001  start=0  InitialOutput=0
  Saturation : Saturate  UpperLimit=1  LowerLimit=0.9646
  Scope : Scope
  Scope7 : Scope  NumInputPorts=5
  Scope8 : Scope  NumInputPorts=6
  Scope9 : Scope  NumInputPorts=2
  Step1 : Step  Time=8  Before=0.9646  After=0.9646  SampleTime=0
  Synchronous Machine pu Standard3 : spsSynchronousMachinepuStandardLib/Synchronous Machine pu Standard  PresetModel=No  MechanicalLoad=Mechanical power Pm  ShowDetailedParameters=on  RotorType=Round  Units=per unit standard parameters  MeasurementBus=off  NominalParameters=[2200e+06 24000 60]  Reactances1=[ 2.07, 0.28, 0.215, 1.99, 0.49, 0.215, 0.155 ]  Reactances2=[2.07 0.28 0.215 1.99 0.215 0.155]  dAxisTimeConstants=Open-circuit  qAxisTimeConstants=Open-circuit  TimeConstants1="[ 4.1  0.033  0.062  ]"  TimeConstants2=[ 4.1, 0.033 , .56 , 0.062 ]  TimeConstants3="[  4.49  0.0681  0.0513  ]"  TimeConstants4=[ 8.0, 0.03, 0.3371, 0.0295 ]  TimeConstants5=[ 1.01, 0.053, 0.1 ]  TimeConstants6=[ 1.3201, 0.023, 1.0, 0.07 ]  TimeConstants7=[4.1 0.033 0.062]  TimeConstants8=[ 1.3201, 0.0231, 0.3371, 0.0295 ]  StatorResistance=0.0046  Mechanical=[2.09 0 2]  PolePairs=20  InitialConditions=[0 -8.04418 0.928649 0.928649 0.928649 23.4946 -96.5054 143.495 1.69595]  SetSaturation=off  Saturation=[0.6404,0.7127,0.8441,0.9214,0.9956,1.082,1.19,1.316,1.457;0.7,0.7698,0.8872,0.9466,0.9969,1.046,1.1,1.151,1.201]  LoadFlowParameters=[1 1736000000 23150.4 0 0]  TsPowergui=0  TsBlock=-1  IterativeModel=Trapezoidal non iterative  IterativeDiscreteModel=Trapezoidal non iterative  BusType=PV  Pref=1736000000  Qref=0  Qmin=-Inf  Qmax=Inf  PLF=0  QLF=0
  Three-Phase V-I Measurement2 : spsThreePhaseVIMeasurementLib/Three-Phase V-I Measurement  VoltageMeasurement=phase-to-ground  SetLabelV=off  LabelV=Vabc  Vpu=on  VpuLL=off  CurrentMeasurement=yes  SetLabelI=off  LabelI=Iabc  Ipu=on  Pbase=2200e6  Vbase=24e3  OutputType=Magnitude  PhasorSimulation=on  PSBequivalent=0
  a : PMIOPort  Side=Right
  b : PMIOPort  Port=2  Side=Right
  c : PMIOPort  Port=3  Side=Right
  tag scope: G2_Ifd=global, G2_Q2=global
  wires:
  Three-Phase V-I Measurement2/1 -> Scope7/5
  Bus Selector6/1 -> Scope8/4, Excitation System3/3  "<Stator voltage  vd (pu)>"
  Bus Selector6/2 -> Scope8/6, Excitation System3/2  "<Stator voltage  vq (pu)>"
  Synchronous Machine pu Standard3/1 -> Bus Selector5/1, Bus Selector6/1
  Hydraulic Turbine and Governor3/1 -> Synchronous Machine pu Standard3/1
  Three-Phase V-I Measurement2/2 -> Scope7/4
  Bus Selector5/6 -> Scope7/3  "<Stator current>"
  Bus Selector6/4 -> Scope8/2, Hydraulic Turbine and Governor3/4  "<Output active power   Peo (pu)>"
  Saturation/1 -> Scope/1
  Ground3/1 -> Excitation System3/4
  Excitation System3/1 -> Synchronous Machine pu Standard3/2, Scope9/1
  Bus Selector6/3 -> Scope8/5, Hydraulic Turbine and Governor3/5  "<Rotor speed deviation  dw (pu)>"
  Bus Selector6/5 -> Scope8/3, Hydraulic Turbine and Governor3/3  "<Rotor speed  wm  (pu)>"
  Constant3/1 -> Hydraulic Turbine and Governor3/1
  Bus Selector5/5 -> Scope7/2  "<Rotor speed  wm  (pu)>"
  Constant4/1 -> Hydraulic Turbine and Governor3/2
  Bus Selector6/6 -> Scope8/1  "<Stator current>"
  Bus Selector5/7 -> [G2_Q2], Scope7/1  "<Output reactive power  Qeo (pu)>"
  Ramp/1 -> Add/2
  Constant1/1 -> Add/1
  Add/1 -> Saturation/1
  Step1/1 -> Excitation System3/1
  Bus Selector5/1 -> [G2_Ifd]  "<Field current  ifd (pu)>"
  connections:
  Three-Phase V-I Measurement2/RConn3 -- c/RConn1
  a/RConn1 -- Three-Phase V-I Measurement2/RConn1
  Three-Phase V-I Measurement2/LConn2 -- Synchronous Machine pu Standard3/RConn2
  Three-Phase V-I Measurement2/LConn1 -- Synchronous Machine pu Standard3/RConn1
  Three-Phase V-I Measurement2/LConn3 -- Synchronous Machine pu Standard3/RConn3
  b/RConn1 -- Three-Phase V-I Measurement2/RConn2

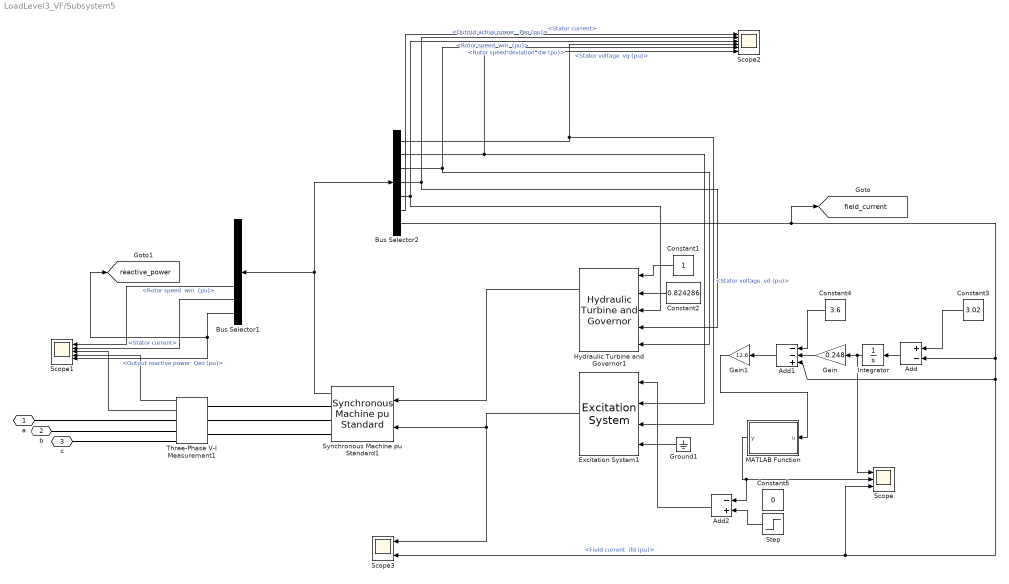
== system LoadLevel3_VF/Subsystem5 ==
  Add : Sum  Inputs=+-
  Add1 : Sum  Inputs=--+
  Add2 : Sum  Inputs=-+
  Bus Selector1 : BusSelector  OutputSignals="dq0 components.Stator voltage  vd (pu),dq0 components.Stator voltage  vq (pu),Mechanical.Rotor speed deviation  dw (pu),Output active power   Peo (pu),Mechanical.Rotor speed  wm  (pu),Stator current,Output reactive power  Qeo (pu)"
  Bus Selector2 : BusSelector  OutputSignals="dq0 components.Stator voltage  vd (pu),dq0 components.Stator voltage  vq (pu),Mechanical.Rotor speed deviation  dw (pu),Output active power   Peo (pu),Mechanical.Rotor speed  wm  (pu),Stator current,dq0 components.Field current  ifd (pu)"
  Constant1 : Constant
  Constant2 : Constant  Value=0.824286
  Constant3 : Constant  Value=3.02
  Constant4 : Constant  Value=3.6
  Constant5 : Constant  Value=0
  Excitation System1 : spsExcitationSystemLib/Excitation System  tr=20e-3  reg=[ 400, 0.02 ]  exc=[ 1, 0 ]  tgr=[ 0, 0 ]  damp=[ 0.001, 0.1 ]  sat=[ 0, 0 ]  lim=[ -11.5, 11.5, 0 ]  v0=[1.04,1.64292]
      settings: LibrarySourceBlock=sps_lib/Electrical Machines/Synchronous Machine Control/Excitation System
  Gain : Gain  Gain=0.248
  Gain1 : Gain  Gain=12.6
  Ground1 : Ground
  Hydraulic Turbine and Governor1 : spsHydraulicTurbineandGovernorLib/Hydraulic Turbine and Governor  sm="[ 10/3  0.07 ]"  gate="[  0.01  0.97518  -0.1  0.1 ]"  reg="[  0.05  1.163  0.105  0  0.01  ]"  hyd="[  0  2.67  ]"  dref=0  po=0.828428
      settings: LibrarySourceBlock=|
      | sps_lib/Electrical Machines/Synchronous Machine Control/Hydraulic Turbine
      | and Governor
  Integrator : Integrator  LimitOutput=on  UpperSaturationLimit=0  LowerSaturationLimit=-3.85
  MATLAB Function : MATLAB Function  TreatAsAtomicUnit=on
  Scope : Scope  NumInputPorts=3
  Scope1 : Scope  NumInputPorts=5
  Scope2 : Scope  NumInputPorts=6
  Scope3 : Scope  NumInputPorts=2
  Step : Step  Time=0  Before=1.04  After=1.04  SampleTime=0
  Synchronous Machine pu Standard1 : spsSynchronousMachinepuStandardLib/Synchronous Machine pu Standard  PresetModel=No  MechanicalLoad=Mechanical power Pm  ShowDetailedParameters=on  RotorType=Round  Units=per unit standard parameters  MeasurementBus=off  NominalParameters=[1400e+06 24000 60]  Reactances1=[2.07 0.28 0.215 1.99 0.49 0.215 0.155]  Reactances2=[2.07 0.28 0.215 1.99 0.215 0.155]  dAxisTimeConstants=Open-circuit  qAxisTimeConstants=Open-circuit  TimeConstants1="[ 4.1  0.033  0.062  ]"  TimeConstants2=[ 4.10 0.033 0.56 0.062 ]  TimeConstants3="[  4.49  0.0681  0.0513  ]"  TimeConstants4=[ 8.0, 0.03, 0.3371, 0.0295 ]  TimeConstants5=[ 1.01, 0.053, 0.1 ]  TimeConstants6=[ 1.3201, 0.023, 1.0, 0.07 ]  TimeConstants7=[4.1 0.033 0.062]  TimeConstants8=[ 1.3201, 0.0231, 0.3371, 0.0295 ]  StatorResistance=0.0046  Mechanical=[2.33 0 2]  PolePairs=20  InitialConditions=[0 -18.5282 0.94897 0.94897 0.94897 15.0201 -104.98 135.02 1.64292]  SetSaturation=off  Saturation=[0.6404,0.7127,0.8441,0.9214,0.9956,1.082,1.19,1.316,1.457;0.7,0.7698,0.8872,0.9466,0.9969,1.046,1.1,1.151,1.201]  LoadFlowParameters=[1 1154000000 24960 0 0]  TsPowergui=0  TsBlock=-1  IterativeModel=Trapezoidal non iterative  IterativeDiscreteModel=Trapezoidal non iterative  BusType=PV  Pref=1154000000  Qref=0  Qmin=-Inf  Qmax=Inf  PLF=0  QLF=0
  Three-Phase V-I Measurement1 : spsThreePhaseVIMeasurementLib/Three-Phase V-I Measurement  VoltageMeasurement=phase-to-ground  SetLabelV=off  LabelV=Vabc  Vpu=on  VpuLL=off  CurrentMeasurement=yes  SetLabelI=off  LabelI=Iabc  Ipu=on  Pbase=1400e6  Vbase=24e3  OutputType=Magnitude  PhasorSimulation=on  PSBequivalent=0
  a : PMIOPort  Side=Right
  b : PMIOPort  Port=2  Side=Right
  c : PMIOPort  Port=3  Side=Right
  tag scope: field_current=global, reactive_power=global
  wires:
  Three-Phase V-I Measurement1/1 -> Scope1/4
  Bus Selector2/1 -> Excitation System1/3, Scope2/4  "<Stator voltage  vd (pu)>"
  Three-Phase V-I Measurement1/2 -> Scope1/3
  Bus Selector2/6 -> Scope2/1  "<Stator current>"
  Hydraulic Turbine and Governor1/1 -> Synchronous Machine pu Standard1/1
  Bus Selector2/3 -> Hydraulic Turbine and Governor1/5, Scope2/5  "<Rotor speed deviation  dw (pu)>"
  Bus Selector2/4 -> Hydraulic Turbine and Governor1/4, Scope2/2  "<Output active power   Peo (pu)>"
  Constant1/1 -> Hydraulic Turbine and Governor1/1
  Bus Selector2/5 -> Hydraulic Turbine and Governor1/3, Scope2/3  "<Rotor speed  wm  (pu)>"
  Excitation System1/1 -> Scope3/1, Synchronous Machine pu Standard1/2
  Constant2/1 -> Hydraulic Turbine and Governor1/2
  Bus Selector2/2 -> Excitation System1/2, Scope2/6  "<Stator voltage  vq (pu)>"
  Bus Selector1/5 -> Scope1/1  "<Rotor speed  wm  (pu)>"
  Synchronous Machine pu Standard1/1 -> Bus Selector2/1, Bus Selector1/1
  Bus Selector1/6 -> Scope1/2  "<Stator current>"
  Ground1/1 -> Excitation System1/4
  Gain1/1 -> MATLAB Function/1(u)
  Constant4/1 -> Add1/1
  Add1/1 -> Gain1/1
  Gain/1 -> Add1/2
  Integrator/1 -> Scope/1, Gain/1
  Constant3/1 -> Add/1
  Add/1 -> Integrator/1
  Step/1 -> Add2/2
  Add2/1 -> Excitation System1/1
  MATLAB Function/1(y) -> Add2/1, Scope/2
  Bus Selector2/7 -> [field_current], Add/2, Add1/3, Scope/3, Scope3/2  "<Field current  ifd (pu)>"
  Bus Selector1/7 -> [reactive_power], Scope1/5  "<Output reactive power  Qeo (pu)>"
  connections:
  Three-Phase V-I Measurement1/RConn1 -- a/RConn1
  Three-Phase V-I Measurement1/LConn2 -- Synchronous Machine pu Standard1/RConn2
  Three-Phase V-I Measurement1/RConn2 -- b/RConn1
  Three-Phase V-I Measurement1/LConn1 -- Synchronous Machine pu Standard1/RConn1
  Three-Phase V-I Measurement1/LConn3 -- Synchronous Machine pu Standard1/RConn3
  Three-Phase V-I Measurement1/RConn3 -- c/RConn1

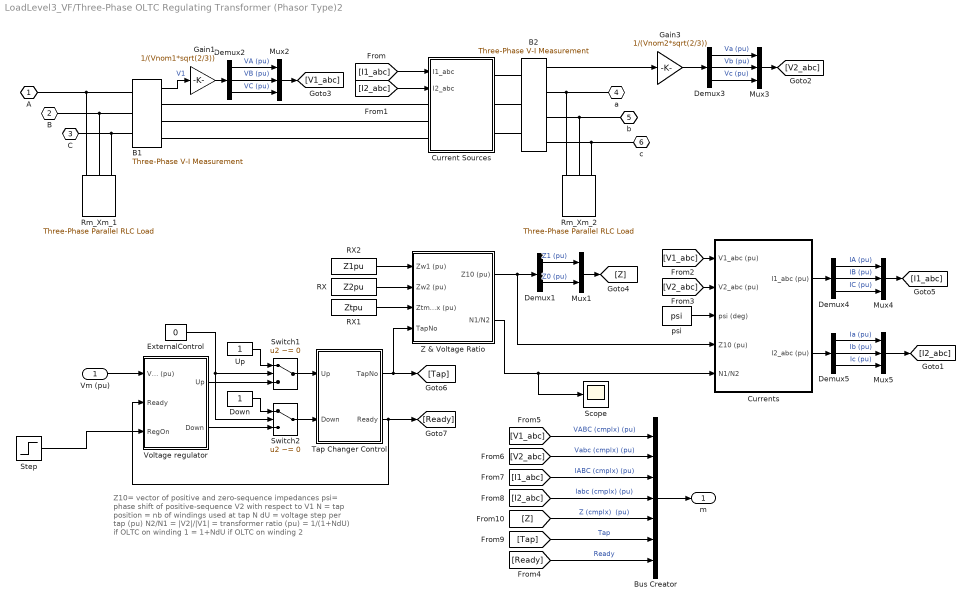
== system LoadLevel3_VF/Three-Phase OLTC Regulating Transformer (Phasor Type)2 ==
  note: Z10= vector of positive and zero-sequence impedances
      | psi= phase shift of positive-sequence V2 with respect to V1
      | N =  tap position = nb of windings used at tap N
      | dU = voltage step  per tap (pu)
      | N2/N1 =  |V2|/|V1| = transformer ratio  (pu)
      |             = 1/(1+NdU)  if OLTC on winding 1
      |             = 1+NdU        if OLTC on winding 2
  Vm (pu) : Inport
  " Currents " : Subsystem
  "B1 " : spsThreePhaseVIMeasurementLib/Three-Phase V-I Measurement  VoltageMeasurement=phase-to-ground  SetLabelV=off  LabelV=Vabc_B21  Vpu=off  VpuLL=off  CurrentMeasurement=no  SetLabelI=off  LabelI=Iabc_B21  Ipu=off  Pbase=10e6  Vbase=25e3  OutputType=Complex  PhasorSimulation=on  PSBequivalent=0
  B2 : spsThreePhaseVIMeasurementLib/Three-Phase V-I Measurement  VoltageMeasurement=phase-to-ground  SetLabelV=off  LabelV=Vabc_B21  Vpu=off  VpuLL=off  CurrentMeasurement=no  SetLabelI=off  LabelI=Iabc_B21  Ipu=off  Pbase=10e6  Vbase=25e3  OutputType=Complex  PhasorSimulation=on  PSBequivalent=0
  Bus Creator : BusCreator  Inputs=7
  Current Sources : Subsystem
  Demux1 : Demux  Outputs=2
      settings: DisplayOption=none
  Demux{2..5} (4 alike) : Demux  Outputs=3
      settings: DisplayOption=none
  Down : Constant
  ExternalControl : Constant  Value=0
  Gain1 : Gain  Gain=1/(Vnom1*sqrt(2/3))  SaturateOnIntegerOverflow=on  OutDataTypeStr=Inherit: Same as input  ParamDataTypeStr=Inherit: Same as input
  Gain3 : Gain  Gain=1/(Vnom2*sqrt(2/3))  SaturateOnIntegerOverflow=on  OutDataTypeStr=Inherit: Same as input  ParamDataTypeStr=Inherit: Same as input
  Mux1 : Mux  Inputs=2
  Mux{2..5} (4 alike) : Mux  Inputs=3
  RX : Constant  Value=Z2pu
  RX1 : Constant  Value=Ztpu
  RX2 : Constant  Value=Z1pu
  Rm_Xm_1 : spsThreePhaseParallelRLCLoadLib/Three-Phase Parallel RLC Load  LConnTagsString=A|B|C  Configuration=Y (grounded)  NominalVoltage=Vnom1  Vabc=[1e3 1e3 1e3]  Vabcp=[1e3 1e3 1e3]  NominalFrequency=Fnom  UnbalancedPower=off  ActivePower=Pnom/RmXm(1)/2  InductivePower=Pnom/RmXm(2)/2  CapacitivePower=0  Pabc=[10e3 9e3 11e3]  QLabc=[100 90 110]  QCabc=[100 90 110]  Pabcp=[10e3 9e3 11e3]  QLabcp=[100 90 110]  QCabcp=[100 90 110]  Measurements=None  LoadType=constant Z
  Rm_Xm_2 : spsThreePhaseParallelRLCLoadLib/Three-Phase Parallel RLC Load  LConnTagsString=A|B|C  Configuration=Y (grounded)  NominalVoltage=Vnom2  Vabc=[1e3 1e3 1e3]  Vabcp=[1e3 1e3 1e3]  NominalFrequency=Fnom  UnbalancedPower=off  ActivePower=Pnom/RmXm(1)/2  InductivePower=Pnom/RmXm(2)/2  CapacitivePower=0  Pabc=[10e3 9e3 11e3]  QLabc=[100 90 110]  QCabc=[100 90 110]  Pabcp=[10e3 9e3 11e3]  QLabcp=[100 90 110]  QCabcp=[100 90 110]  Measurements=None  LoadType=constant Z
  Scope : Scope
  Step : Step  Time=40  After=RegulatorOn  SampleTime=0
  Switch1 : Switch  Criteria=u2 ~= 0  SaturateOnIntegerOverflow=off  InputSameDT=off
  Switch2 : Switch  Criteria=u2 ~= 0  SaturateOnIntegerOverflow=off  InputSameDT=off
  Tap Changer Control : Subsystem  mask(Tap Changer Control){MinMaxTap=TapMinMax, InitialPosition=InitialTap, MecDelay=TapSelectionTime}
      mask prompts: MinMaxTap "Minimum and maximum tap number [ Min  Max ] :"; InitialPosition "Initial tap position"; MecDelay "Mechanical delay time"
      mask init:
      | if MecDelay<=0,
      | 	MecDelay=1/60;
      | end
  Up : Constant
  Voltage regulator : Subsystem  mask{Vref=RegulatorVref, DeadBand=RegulatorDeadBand, TimeDelay=RegulatorDelay}
      mask prompts: Vref "Vref (pu)"; DeadBand "Deadband (pu)"; TimeDelay "Time delay (s)"
  Z & Voltage Ratio : Subsystem
  psi : Constant  Value=psi
  A : PMIOPort  Tag=PMCPort  Side=Left
  B : PMIOPort  Tag=PMCPort  Port=2  Side=Left
  C : PMIOPort  Tag=PMCPort  Port=3  Side=Left
  a : PMIOPort  Tag=PMCPort  Port=4  Side=Right
  b : PMIOPort  Tag=PMCPort  Port=5  Side=Right
  c : PMIOPort  Tag=PMCPort  Port=6  Side=Right
  m : Outport  VectorParamsAs1DForOutWhenUnconnected=off
  wires:
  [Ready] -> Bus Creator/7  "Ready"
  Step/1 -> Voltage regulator/3(RegOn)
  Switch2/1 -> Tap Changer Control/2("Down ")
  ExternalControl/1 -> Switch2/2, Switch1/2
  Down/1 -> Switch2/1
  Up/1 -> Switch1/1
  Switch1/1 -> Tap Changer Control/1("Up ")
  Voltage regulator/2("Down ") -> Switch2/3
  Voltage regulator/1("Up ") -> Switch1/3
  Vm (pu)/1 -> Voltage regulator/1(Vmes (pu))
  Tap Changer Control/2(Ready) -> [Ready], Voltage regulator/2(Ready)
  Tap Changer Control/1(TapNo) -> Z & Voltage Ratio/4(TapNo), [Tap]
  "B1 "/1 -> Gain1/1  "V1"
  RX/1 -> Z & Voltage Ratio/2(Zw2 (pu))
  RX1/1 -> Z & Voltage Ratio/3(Ztmax (pu))
  Z & Voltage Ratio/1("Z10 (pu) ") -> Demux1/1, " Currents "/4(Z10 (pu))
  RX2/1 -> Z & Voltage Ratio/1(Zw1 (pu))
  Z & Voltage Ratio/2(N1/N2) -> Scope/1, " Currents "/5(N1/N2)
  [I1_abc] -> Current Sources/1(I1_abc)
  [I2_abc] -> Current Sources/2(I2_abc)
  B2/1 -> Gain3/1
  Gain3/1 -> Demux3/1
  Gain1/1 -> Demux2/1
  [V1_abc] -> " Currents "/1(V1_abc (pu))
  [V2_abc] -> " Currents "/2(V2_abc (pu))
  psi/1 -> " Currents "/3(psi (deg))
  [V2_abc] -> Bus Creator/2  "Vabc (cmplx) (pu)"
  Bus Creator/1 -> m/1
  [I1_abc] -> Bus Creator/3  "IABC (cmplx) (pu)"
  [I2_abc] -> Bus Creator/4  "Iabc (cmplx) (pu)"
  [Tap] -> Bus Creator/6  "Tap"
  Demux1/1 -> Mux1/1  "Z1 (pu)"
  Demux1/2 -> Mux1/2  "Z0 (pu)"
  Mux1/1 -> [Z]
  [Z] -> Bus Creator/5  "Z (cmplx)  (pu)"
  Demux2/1 -> Mux2/1  "VA (pu)"
  Demux2/2 -> Mux2/2  "VB (pu)"
  Demux2/3 -> Mux2/3  "VC (pu)"
  Mux2/1 -> [V1_abc]
  [V1_abc] -> Bus Creator/1  "VABC (cmplx) (pu)"
  Demux3/1 -> Mux3/1  "Va (pu)"
  Demux3/2 -> Mux3/2  "Vb (pu)"
  Demux3/3 -> Mux3/3  "Vc (pu)"
  Mux3/1 -> [V2_abc]
  Demux4/1 -> Mux4/1  "IA (pu)"
  Demux4/2 -> Mux4/2  "IB (pu)"
  Demux4/3 -> Mux4/3  "IC (pu)"
  Mux4/1 -> [I1_abc]
  " Currents "/1(I1_abc (pu)) -> Demux4/1
  Demux5/1 -> Mux5/1  "Ia (pu)"
  Demux5/2 -> Mux5/2  "Ib (pu)"
  Demux5/3 -> Mux5/3  "Ic (pu)"
  Mux5/1 -> [I2_abc]
  " Currents "/2("I2_abc (pu) ") -> Demux5/1
  connections:
  Current Sources/RConn3 -- B2/LConn3
  Current Sources/RConn2 -- B2/LConn2
  Current Sources/RConn1 -- B2/LConn1
  "B1 "/RConn3 -- Current Sources/LConn3
  "B1 "/RConn2 -- Current Sources/LConn2
  Current Sources/LConn1 -- "B1 "/RConn1
  A/RConn1 -- "B1 "/LConn1 -- Rm_Xm_1/LConn1
  B/RConn1 -- "B1 "/LConn2 -- Rm_Xm_1/LConn2
  C/RConn1 -- "B1 "/LConn3 -- Rm_Xm_1/LConn3
  c/RConn1 -- B2/RConn3 -- Rm_Xm_2/LConn3
  b/RConn1 -- B2/RConn2 -- Rm_Xm_2/LConn2
  a/RConn1 -- B2/RConn1 -- Rm_Xm_2/LConn1
